simulink model "netra_telemedicine"  (R2026a)
settings: Solver=VariableStepAuto  StopTime=2592000
model workspace (MAT data in the model file):
  ai_time = 30
  mean_arrival = 315
  num_reviewers = 3
  review_time = 180
  upload_time = 1.6
values from neighbouring files (symbols this model uses):
  n = numel(arr)    [queueSim.m]
undefined symbols (not defined in the file or in its folder): m
settings Model: Creator=sharm  LastModifiedBy=sharm

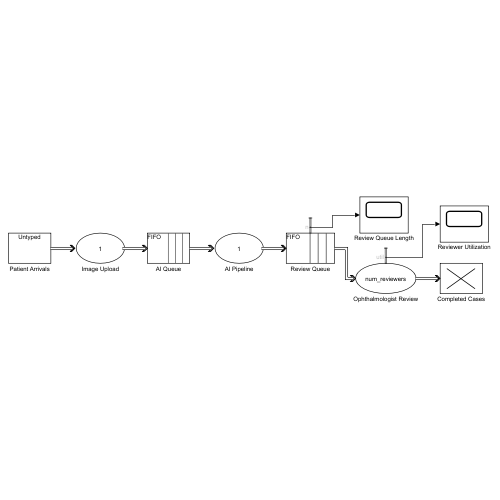
[thumbnail: Simulink's stored preview of the top-level diagram]
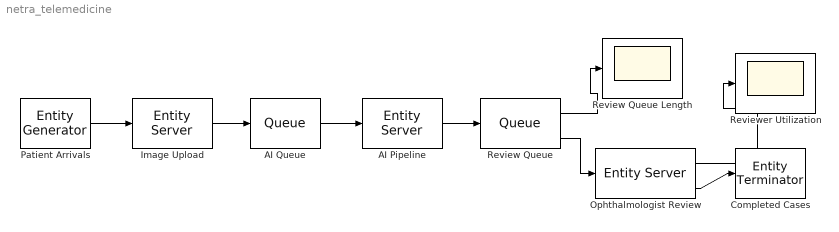
== system netra_telemedicine ==
  AI Pipeline : EntityServer  InputPortMessageModes=m  OutputPortMessageModes=m  Capacity=1  ServiceTimeValue=ai_time
  AI Queue : Queue  InputPortMessageModes=m  OutputPortMessageModes=m  Capacity=inf
  Completed Cases : EntityTerminator  InputPortMessageModes=m
  Image Upload : EntityServer  InputPortMessageModes=m  OutputPortMessageModes=m  Capacity=1  ServiceTimeValue=upload_time
  Ophthalmologist Review : EntityServer  InputPortMessageModes=m  OutputPortMessageModes=n,m  Capacity=num_reviewers  ServiceTimeValue=review_time  Utilization=on
      settings: OutputPortMap=o5,o9
  Patient Arrivals : EntityGenerator  OutputPortMessageModes=m  Period=mean_arrival  EntityTypeName=Entity
  Review Queue : Queue  InputPortMessageModes=m  OutputPortMessageModes=n,m  Capacity=inf  NumberEntitiesInBlock=on
      settings: OutputPortMap=o1,o5
  Review Queue Length : Scope
  Reviewer Utilization : Scope
  wires:
  Ophthalmologist Review/2 -> Completed Cases/1
  Ophthalmologist Review/1 -> Reviewer Utilization/1
  Review Queue/2 -> Ophthalmologist Review/1
  Review Queue/1 -> Review Queue Length/1
  AI Pipeline/1 -> Review Queue/1
  AI Queue/1 -> AI Pipeline/1
  Image Upload/1 -> AI Queue/1
  Patient Arrivals/1 -> Image Upload/1
